simulink library "ad_blocks"  (R2017a)
settings: Solver=VariableStepAuto  StartTime=0.0  StopTime=10.0  RelTol=1e-3
undefined symbols (not defined in the file or in its folder): DiscIntNeverNeededParam
undefined symbols (not defined in the file): BatchSize, densesize, features1, features2, filtersize1
libraries: ad_blocks x23, simulink x5, dspindex x2
(part 2 of 2)

== matlab function ad_blocks/softmax_cross_entropy_with_logits/function ==
  data: logits input; loss output; logitsoffsetted output size=size(logits); labels input; sumx output size=size(logits,1)
function [loss,logitsoffsetted,sumx] = fcn(logits,labels)
classes = size(logits,2);
classdim = 2;
logitsmax = max(logits,[],classdim); % batch x 1
            logitsoffsetted = logits - repmat(logitsmax(:),1,classes); % batch x classes
            sumx = sum(exp(logitsoffsetted),classdim); % exp and sum along class: batch x 1
            loss = sum((labels .* (repmat(log(sumx),1,classes) - logitsoffsetted)),classdim);

== matlab function ad_blocks/softmax_cross_entropy_with_logits/gradient ==
  data: logits input; J output size=size(logits); labels input; Jin input; logitsoffsetted input; sumx input
function J  = fcn(logits,labels,Jin,logitsoffsetted,sumx)

% output = batch x 1
% logits = batch x C
classes = size(logits,2);
a = (exp(logitsoffsetted) ./ repmat(sumx,1,classes)); % batch x 1 WHY?
Jo = a-labels; % batch x C
J = repmat(Jin,1,classes).*Jo;

== matlab function ad_blocks/Softmax AD/MATLAB Function1 ==
  data: u input; y output
function y = fcn(u)
%#codegen
exps = exp(u-max(u(:)));
y = exps/sum(exps(:));

== matlab function ad_blocks/Softmax AD/MATLAB Function2 ==
  data: u input; y output
function y = fcn(u)

y = 1./(1+exp(-u));

== matlab function ad_blocks/Adam Old/MATLAB Function ==
  data: lrt input size=1; y output size=size(m_t); m_t input; s_t input; epsilon input size=1
function y = fcn(lrt,m_t,s_t,epsilon)

y =lrt * m_t ./ (sqrt(s_t) + epsilon);

== matlab function ad_blocks/Adam Old/Moment Update/MATLAB Function ==
  data: u input; y output
function y = fcn(u)

y = 1-u;

== matlab function ad_blocks/Adam Old/Second Moment Update/MATLAB Function ==
  data: u input; y output
function y = fcn(u)

y = 1-u;

== matlab function ad_blocks/Adam as Gradient/Adam Rate1/MATLAB Function ==
  data: learningrate input; ltr output; beta1 input; beta2 input; t input
function ltr = fcn(learningrate,beta1,beta2,t)

if beta1 == 1 || beta2 == 1
    ltr = -learningrate;
else
    ltr = - learningrate * sqrt(1 - beta2^t) / (1 - beta1^t);
end

== matlab function ad_blocks/Size ==
  data: u input; n output; s output
function [n,s] = fcn(u)

n = ndims(u);
s = [size(u,1) size(u,2) size(u,3) size(u,4)];
